simulink model "GUAM"  (R2023b)
settings: Solver=FixedStepAuto  StartTime=0.0  StopTime=SimIn.stopTime  FixedStep=Ts  RelTol=1e-3  AbsTol=1e-4  EnableMultiTasking=on
PostLoadFcn:
  | warning('off','sm:sli:setup:compile:LocalSolverNotSupported')
StartFcn:
  | tic
StopFcn:
  | Elapsed_Sim_Time = toc;
model workspace: external: MATLAB File aileronAssembly_DataFile.m (data not in the file)
values from neighbouring files (symbols this model uses):
  Ts = 0.05    [RUNME.m]
undefined symbols (not defined in the file or in its folder): AAC_Param, ang2Ext_coeff, Ki, Ki_scaling_elec, Kp, Leadscrew, motor_friction, R7_sctrl, sigbuilder_block, SimIn, SimPar, sm_aileron_actuator_lib, smiData, X, Y, Z
libraries: sm_lib x608, fl_lib x378, ee_lib x105, nesl_utility x96, simulink x10, eeGeneralControl x7, sh_lib x7, dspstat3 x6, sdl_lib x3, slpidlib x2, aerolibfltsims x2
(part 2 of 22)

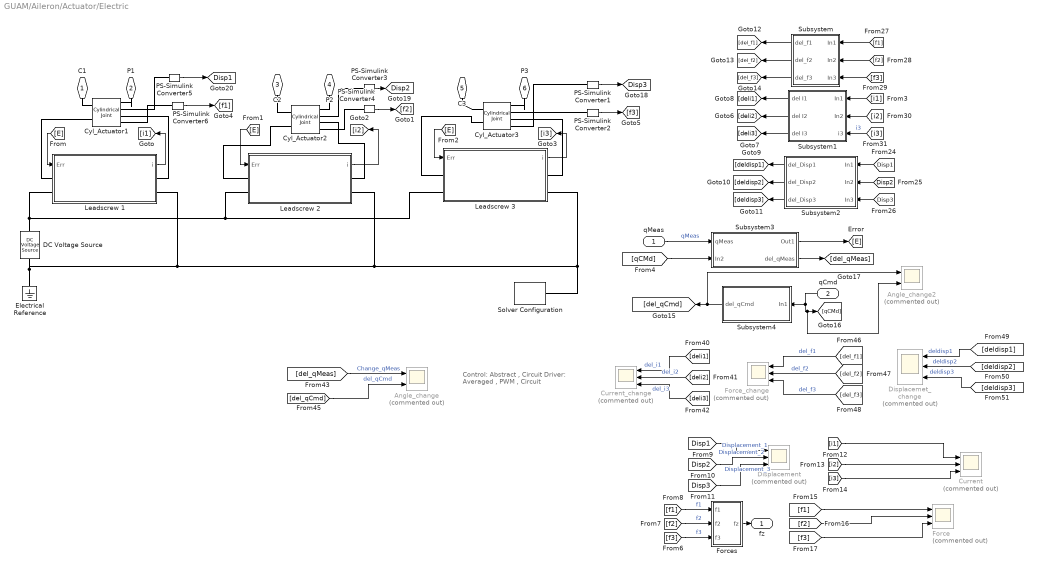
== system GUAM/Aileron/Actuator/Electric ==
  note: Control: Abstract , Circuit
      | Driver: Averaged , PWM , Circuit
  qMeas : Inport
  "qCmd " : Inport  Port=2
  Angle_change : Scope  Commented=on  NumInputPorts=2
  Angle_change2 : Scope  Commented=on  NumInputPorts=2
  Current : Scope  Commented=on  NumInputPorts=3
  Current_change : Scope  Commented=on  NumInputPorts=3
  Cyl_Actuator1 : sm_lib/Joints/Cylindrical Joint  JointMode=Normal  SenseConstraintForce=off  SenseConstraintForceX=off  SenseConstraintForceY=off  SenseConstraintForceZ=off  SenseConstraintTorque=off  SenseConstraintTorqueX=off  SenseConstraintTorqueY=off  SenseConstraintTorqueZ=off  SenseTotalForce=off  SenseTotalForceX=off  SenseTotalForceY=off  SenseTotalForceZ=off  SenseTotalTorque=off  SenseTotalTorqueX=off  SenseTotalTorqueY=off  SenseTotalTorqueZ=off  CompositeWrenchDir=FollowerOnBase  CompositeWrenchFrame=BaseFrame  PzEquilibriumPosition=AAC_Param.Act.El.Spr.l0  PzEquilibriumPositionUnits=m  PzSpringStiffness=AAC_Param.Act.El.Spr.k  PzSpringStiffnessUnits=N/m  PzDampingCoefficient=AAC_Param.Act.El.Spr.b  PzDampingCoefficientUnits=N/(m/s)  PzTorqueActuationMode=InputTorque  PzMotionActuationMode=ComputedMotion  PzSensePosition=on  PzSenseVelocity=on  PzSenseAcceleration=off  PzSenseTorqueForce=on  PzSenseLowerLimitTorqueForce=off  PzSenseUpperLimitTorqueForce=off  PzLowerLimitSpecify=off  PzLowerLimitBound=-1  PzLowerLimitBoundUnits=m  PzLowerLimitStiffness=1e6  PzLowerLimitStiffnessUnits=N/m  PzLowerLimitDamping=1e3  PzLowerLimitDampingUnits=N/(m/s)  PzLowerLimitTransitionRegionWidth=1e-4  PzLowerLimitTransitionRegionWidthUnits=m  PzUpperLimitSpecify=off  PzUpperLimitBound=1  PzUpperLimitBoundUnits=m  PzUpperLimitStiffness=1e6  PzUpperLimitStiffnessUnits=N/m  PzUpperLimitDamping=1e3  PzUpperLimitDampingUnits=N/(m/s)  PzUpperLimitTransitionRegionWidth=1e-4  PzUpperLimitTransitionRegionWidthUnits=m  PzPositionTargetSpecify=on  PzPositionTargetPriority=Low  PzPositionTargetValue=smiData.CylindricalJoint(3).Pz.Pos  PzPositionTargetValueUnits=m  PzVelocityTargetSpecify=off  PzVelocityTargetPriority=High  PzVelocityTargetValue=0  PzVelocityTargetValueUnits=m/s  RzEquilibriumPosition=0  RzEquilibriumPositionUnits=rad  RzSpringStiffness=0  RzSpringStiffnessUnits=N*m/rad  RzDampingCoefficient=0  RzDampingCoefficientUnits=N*m/(rad/s)  RzTorqueActuationMode=NoTorque  RzMotionActuationMode=ComputedMotion  RzSensePosition=off  RzSenseVelocity=off  RzSenseAcceleration=off  RzSenseTorqueForce=off  RzSenseLowerLimitTorqueForce=off  RzSenseUpperLimitTorqueForce=off  RzLowerLimitSpecify=off  RzLowerLimitBound=-90  RzLowerLimitBoundUnits=deg  RzLowerLimitStiffness=1e4  RzLowerLimitStiffnessUnits=N*m/deg  RzLowerLimitDamping=10  RzLowerLimitDampingUnits=N*m/(deg/s)  RzLowerLimitTransitionRegionWidth=0.1  RzLowerLimitTransitionRegionWidthUnits=deg  RzUpperLimitSpecify=off  RzUpperLimitBound=90  RzUpperLimitBoundUnits=deg  RzUpperLimitStiffness=1e4  RzUpperLimitStiffnessUnits=N*m/deg  RzUpperLimitDamping=10  RzUpperLimitDampingUnits=N*m/(deg/s)  RzUpperLimitTransitionRegionWidth=0.1  RzUpperLimitTransitionRegionWidthUnits=deg  RzPositionTargetSpecify=on  RzPositionTargetPriority=Low  RzPositionTargetValue=smiData.CylindricalJoint(3).Rz.Pos  RzPositionTargetValueUnits=deg  RzVelocityTargetSpecify=off  RzVelocityTargetPriority=High  RzVelocityTargetValue=0  RzVelocityTargetValueUnits=deg/s
  Cyl_Actuator2 : sm_lib/Joints/Cylindrical Joint  JointMode=Normal  SenseConstraintForce=off  SenseConstraintForceX=off  SenseConstraintForceY=off  SenseConstraintForceZ=off  SenseConstraintTorque=off  SenseConstraintTorqueX=off  SenseConstraintTorqueY=off  SenseConstraintTorqueZ=off  SenseTotalForce=off  SenseTotalForceX=off  SenseTotalForceY=off  SenseTotalForceZ=off  SenseTotalTorque=off  SenseTotalTorqueX=off  SenseTotalTorqueY=off  SenseTotalTorqueZ=off  CompositeWrenchDir=FollowerOnBase  CompositeWrenchFrame=BaseFrame  PzEquilibriumPosition=AAC_Param.Act.El.Spr.l0  PzEquilibriumPositionUnits=m  PzSpringStiffness=AAC_Param.Act.El.Spr.k  PzSpringStiffnessUnits=N/m  PzDampingCoefficient=AAC_Param.Act.El.Spr.b  PzDampingCoefficientUnits=N/(m/s)  PzTorqueActuationMode=InputTorque  PzMotionActuationMode=ComputedMotion  PzSensePosition=on  PzSenseVelocity=on  PzSenseAcceleration=off  PzSenseTorqueForce=on  PzSenseLowerLimitTorqueForce=off  PzSenseUpperLimitTorqueForce=off  PzLowerLimitSpecify=off  PzLowerLimitBound=-1  PzLowerLimitBoundUnits=m  PzLowerLimitStiffness=1e6  PzLowerLimitStiffnessUnits=N/m  PzLowerLimitDamping=1e3  PzLowerLimitDampingUnits=N/(m/s)  PzLowerLimitTransitionRegionWidth=1e-4  PzLowerLimitTransitionRegionWidthUnits=m  PzUpperLimitSpecify=on  PzUpperLimitBound=1  PzUpperLimitBoundUnits=m  PzUpperLimitStiffness=1e6  PzUpperLimitStiffnessUnits=N/m  PzUpperLimitDamping=1e3  PzUpperLimitDampingUnits=N/(m/s)  PzUpperLimitTransitionRegionWidth=1e-4  PzUpperLimitTransitionRegionWidthUnits=m  PzPositionTargetSpecify=on  PzPositionTargetPriority=Low  PzPositionTargetValue=smiData.CylindricalJoint(2).Pz.Pos  PzPositionTargetValueUnits=m  PzVelocityTargetSpecify=off  PzVelocityTargetPriority=High  PzVelocityTargetValue=0  PzVelocityTargetValueUnits=m/s  RzEquilibriumPosition=0  RzEquilibriumPositionUnits=rad  RzSpringStiffness=0  RzSpringStiffnessUnits=N*m/rad  RzDampingCoefficient=0  RzDampingCoefficientUnits=N*m/(rad/s)  RzTorqueActuationMode=NoTorque  RzMotionActuationMode=ComputedMotion  RzSensePosition=off  RzSenseVelocity=off  RzSenseAcceleration=off  RzSenseTorqueForce=off  RzSenseLowerLimitTorqueForce=off  RzSenseUpperLimitTorqueForce=off  RzLowerLimitSpecify=off  RzLowerLimitBound=-90  RzLowerLimitBoundUnits=deg  RzLowerLimitStiffness=1e4  RzLowerLimitStiffnessUnits=N*m/deg  RzLowerLimitDamping=10  RzLowerLimitDampingUnits=N*m/(deg/s)  RzLowerLimitTransitionRegionWidth=0.1  RzLowerLimitTransitionRegionWidthUnits=deg  RzUpperLimitSpecify=off  RzUpperLimitBound=90  RzUpperLimitBoundUnits=deg  RzUpperLimitStiffness=1e4  RzUpperLimitStiffnessUnits=N*m/deg  RzUpperLimitDamping=10  RzUpperLimitDampingUnits=N*m/(deg/s)  RzUpperLimitTransitionRegionWidth=0.1  RzUpperLimitTransitionRegionWidthUnits=deg  RzPositionTargetSpecify=on  RzPositionTargetPriority=Low  RzPositionTargetValue=smiData.CylindricalJoint(2).Rz.Pos  RzPositionTargetValueUnits=deg  RzVelocityTargetSpecify=off  RzVelocityTargetPriority=High  RzVelocityTargetValue=0  RzVelocityTargetValueUnits=deg/s
  Cyl_Actuator3 : sm_lib/Joints/Cylindrical Joint  JointMode=Normal  SenseConstraintForce=off  SenseConstraintForceX=off  SenseConstraintForceY=off  SenseConstraintForceZ=off  SenseConstraintTorque=off  SenseConstraintTorqueX=off  SenseConstraintTorqueY=off  SenseConstraintTorqueZ=off  SenseTotalForce=off  SenseTotalForceX=off  SenseTotalForceY=off  SenseTotalForceZ=off  SenseTotalTorque=off  SenseTotalTorqueX=off  SenseTotalTorqueY=off  SenseTotalTorqueZ=off  CompositeWrenchDir=FollowerOnBase  CompositeWrenchFrame=BaseFrame  PzEquilibriumPosition=AAC_Param.Act.El.Spr.l0  PzEquilibriumPositionUnits=m  PzSpringStiffness=AAC_Param.Act.El.Spr.k  PzSpringStiffnessUnits=N/m  PzDampingCoefficient=AAC_Param.Act.El.Spr.b  PzDampingCoefficientUnits=N/(m/s)  PzTorqueActuationMode=InputTorque  PzMotionActuationMode=ComputedMotion  PzSensePosition=on  PzSenseVelocity=on  PzSenseAcceleration=off  PzSenseTorqueForce=on  PzSenseLowerLimitTorqueForce=off  PzSenseUpperLimitTorqueForce=off  PzLowerLimitSpecify=off  PzLowerLimitBound=0  PzLowerLimitBoundUnits=m  PzLowerLimitStiffness=1e6  PzLowerLimitStiffnessUnits=N/m  PzLowerLimitDamping=1e3  PzLowerLimitDampingUnits=N/(m/s)  PzLowerLimitTransitionRegionWidth=0.01  PzLowerLimitTransitionRegionWidthUnits=m  PzUpperLimitSpecify=off  PzUpperLimitBound=0.04  PzUpperLimitBoundUnits=m  PzUpperLimitStiffness=1e6  PzUpperLimitStiffnessUnits=N/m  PzUpperLimitDamping=1e3  PzUpperLimitDampingUnits=N/(m/s)  PzUpperLimitTransitionRegionWidth=1e-4  PzUpperLimitTransitionRegionWidthUnits=m  PzPositionTargetSpecify=on  PzPositionTargetPriority=Low  PzPositionTargetValue=smiData.CylindricalJoint(1).Pz.Pos  PzPositionTargetValueUnits=m  PzVelocityTargetSpecify=off  PzVelocityTargetPriority=High  PzVelocityTargetValue=0  PzVelocityTargetValueUnits=m/s  RzEquilibriumPosition=0  RzEquilibriumPositionUnits=rad  RzSpringStiffness=0  RzSpringStiffnessUnits=N*m/rad  RzDampingCoefficient=0  RzDampingCoefficientUnits=N*m/(rad/s)  RzTorqueActuationMode=NoTorque  RzMotionActuationMode=ComputedMotion  RzSensePosition=off  RzSenseVelocity=off  RzSenseAcceleration=off  RzSenseTorqueForce=off  RzSenseLowerLimitTorqueForce=off  RzSenseUpperLimitTorqueForce=off  RzLowerLimitSpecify=off  RzLowerLimitBound=-90  RzLowerLimitBoundUnits=deg  RzLowerLimitStiffness=1e4  RzLowerLimitStiffnessUnits=N*m/deg  RzLowerLimitDamping=10  RzLowerLimitDampingUnits=N*m/(deg/s)  RzLowerLimitTransitionRegionWidth=0.1  RzLowerLimitTransitionRegionWidthUnits=deg  RzUpperLimitSpecify=off  RzUpperLimitBound=90  RzUpperLimitBoundUnits=deg  RzUpperLimitStiffness=1e4  RzUpperLimitStiffnessUnits=N*m/deg  RzUpperLimitDamping=10  RzUpperLimitDampingUnits=N*m/(deg/s)  RzUpperLimitTransitionRegionWidth=0.1  RzUpperLimitTransitionRegionWidthUnits=deg  RzPositionTargetSpecify=on  RzPositionTargetPriority=Low  RzPositionTargetValue=smiData.CylindricalJoint(1).Rz.Pos  RzPositionTargetValueUnits=deg  RzVelocityTargetSpecify=off  RzVelocityTargetPriority=High  RzVelocityTargetValue=0  RzVelocityTargetValueUnits=deg/s
  DC Voltage Source : fl_lib/Electrical/Electrical Sources/DC Voltage Source  v0=24 V
  Displacement : Scope  Commented=on  NumInputPorts=3
  Displacemet_change : Scope  Commented=on  NumInputPorts=3
  Electrical Reference : fl_lib/Electrical/Electrical Elements/Electrical Reference
  Force : Scope  Commented=on  NumInputPorts=3
  Force_change : Scope  Commented=on  NumInputPorts=3
  Forces : Subsystem
  Leadscrew 1 : Subsystem  AncestorBlock=sm_aileron_actuator_lib/Leadscrew  mask{popup_ctrl=Simulink, popup_driver=Averaged}
      mask prompts: popup_ctrl "Controller"; popup_driver "Driver Circuit"
      mask init:
      | if(popup_ctrl == 1)
      |     set_param([gcb '/Control'],'OverrideUsingVariant','Simulink')
      | else
      |     set_param([gcb '/Control'],'OverrideUsingVariant','Circuit')
      | end
      | 
      | if(popup_driver == 3)
      |     set_param([gcb '/Motor Driver'],'OverrideUsingVariant','Circuit')
      | else
      |     set_param([gcb '/Motor Driver'],'OverrideUsingVariant','Abstract')
      |     if(popup_driver == 1)
      |         set_param([gcb '/Motor Driver/Abstract/Controlled PWM Voltage'],'pwm_or_av','2');
      |         set_param([gcb '/Motor Driver/Abstract/H-Bridge'],'pwm_or_av','2');
      |     else
      |         set_param([gcb '/Motor Driver/Abstract/Controlled PWM Voltage'],'pwm_or_av','1');
      |         set_param([gcb '/Motor Driver/Abstract/H-Bridge'],'pwm_or_av','1');
      |     end
      | end
      | 
      | set_param([gcb '/Control'],'Name','Control');
      | set_param([gcb '/Motor Driver'],'Name','Motor Driver');
      mask TypeOptions popup_ctrl: Simulink | Circuit
      mask TypeOptions popup_driver: Averaged | PWM | Circuit
      mask Display:
      | SnC_Char = get_param(gcb,'popup_ctrl');
      | PWM_Char = get_param(gcb,'popup_driver');
      | 
      | try
      |     image(['sm_aileron_actuator_msc' upper(SnC_Char(1)) 'pw' PWM_Char(1) '_IMAGE.png']);
      | catch
      | 
      | end
  Leadscrew 2 : Subsystem  AncestorBlock=sm_aileron_actuator_lib/Leadscrew  mask{popup_ctrl=Simulink, popup_driver=Averaged}
      mask prompts: popup_ctrl "Controller"; popup_driver "Driver Circuit"
      mask init: same as GUAM/Aileron/Actuator/Electric/Leadscrew 1
      mask TypeOptions popup_ctrl: Simulink | Circuit
      mask TypeOptions popup_driver: Averaged | PWM | Circuit
      mask Display:
      | SnC_Char = get_param(gcb,'popup_ctrl');
      | PWM_Char = get_param(gcb,'popup_driver');
      | 
      | try
      |     image(['sm_aileron_actuator_msc' upper(SnC_Char(1)) 'pw' PWM_Char(1) '_IMAGE.png']);
      | catch
      | 
      | end
  Leadscrew 3 : Subsystem  AncestorBlock=sm_aileron_actuator_lib/Leadscrew  mask{popup_ctrl=Simulink, popup_driver=Averaged}
      mask prompts: popup_ctrl "Controller"; popup_driver "Driver Circuit"
      mask init: same as GUAM/Aileron/Actuator/Electric/Leadscrew 1
      mask TypeOptions popup_ctrl: Simulink | Circuit
      mask TypeOptions popup_driver: Averaged | PWM | Circuit
      mask Display:
      | SnC_Char = get_param(gcb,'popup_ctrl');
      | PWM_Char = get_param(gcb,'popup_driver');
      | 
      | try
      |     image(['sm_aileron_actuator_msc' upper(SnC_Char(1)) 'pw' PWM_Char(1) '_IMAGE.png']);
      | catch
      | 
      | end
  PS-Simulink Converter1 : nesl_utility/PS-Simulink Converter  PhysicalDomain=network_engine_domain  SubClassName=ps_output  LeftPortType=input  RightPortType=output  PseudoPeriodic=off  Frequencies=[]  VectorFormat=1-D array  Unit=m  AffineConversion=off
  PS-Simulink Converter2 : nesl_utility/PS-Simulink Converter  PhysicalDomain=network_engine_domain  SubClassName=ps_output  LeftPortType=input  RightPortType=output  PseudoPeriodic=off  Frequencies=[]  VectorFormat=1-D array  Unit=N  AffineConversion=off
  PS-Simulink Converter3 : nesl_utility/PS-Simulink Converter  PhysicalDomain=network_engine_domain  SubClassName=ps_output  LeftPortType=input  RightPortType=output  PseudoPeriodic=off  Frequencies=[]  VectorFormat=1-D array  Unit=m  AffineConversion=off
  PS-Simulink Converter4 : nesl_utility/PS-Simulink Converter  PhysicalDomain=network_engine_domain  SubClassName=ps_output  LeftPortType=input  RightPortType=output  PseudoPeriodic=off  Frequencies=[]  VectorFormat=1-D array  Unit=N  AffineConversion=off
  PS-Simulink Converter5 : nesl_utility/PS-Simulink Converter  PhysicalDomain=network_engine_domain  SubClassName=ps_output  LeftPortType=input  RightPortType=output  PseudoPeriodic=off  Frequencies=[]  VectorFormat=1-D array  Unit=m  AffineConversion=off
  PS-Simulink Converter6 : nesl_utility/PS-Simulink Converter  PhysicalDomain=network_engine_domain  SubClassName=ps_output  LeftPortType=input  RightPortType=output  PseudoPeriodic=off  Frequencies=[]  VectorFormat=1-D array  Unit=N  AffineConversion=off
  Solver Configuration : nesl_utility/Solver Configuration  PhysicalDomain=network_engine_domain  SubClassName=solver  LeftPortType=input  RightPortType=generic  Tones=[]  Harmonics=[]  SimulateNoise=off  Profile=off  UseLocalSampling=off  EnableSwitchedLinearOptims=on  FrequencyDomain=off  UseCCode=off  RelTol=0.001  AbsTol=0.001  MinStep=1e-09  ToWorkspace=off  RevertToSquareIcSolve=off  NumHomotopyIterations=100  PhasorMode=off  PhasorModeNumHarmonics=1  ConsistencySolver=NEWTON_XTOL_AFTER_FTOL  IndexReductionMethod=DerivativeReplacement  DoDC=off  ResidualTolerance=1e-09  ConsistencyTolSource=GLOBAL  ConsistencyAbsTol=0.001  ConsistencyRelTol=0.001  ConsistencyTolFactor=0.0001  UseLocalSolver=off  LocalSolverChoice=NE_BACKWARD_EULER_ADVANCER  ResolveIndetEquations=on  FunctionEvalNumThread=1  LocalSolverSampleTime=0.001  DoFixedCost=off  MaxNonlinIter=3  MaxModeIter=2  ComputeImpulses=off  ImpulseIterations=2  LinearAlgebra=auto  LinearAlgebraNumThread=0  EquationFormulation=NE_TIME_EF  DelaysMemoryBudget=2048  AutomaticFiltering=on  FilteringTimeConstant=0.001  PartitionStorageMethod=AS_NEEDED  PartitionMemoryBudget=1024  PartitionMethod=ROBUST  MultibodyUseLocalSolver=off  MultibodyLocalSolverChoice=ODE1  MultibodyLocalSolverSampleTime=0.001
  Subsystem : Subsystem
  Subsystem1 : Subsystem
  Subsystem2 : Subsystem
  Subsystem3 : Subsystem
  Subsystem4 : Subsystem
  C1 : PMIOPort  Side=Right
  P1 : PMIOPort  Port=2  Side=Right
  C2 : PMIOPort  Port=3  Side=Right
  P2 : PMIOPort  Port=4  Side=Right
  C3 : PMIOPort  Port=5  Side=Right
  P3 : PMIOPort  Port=6  Side=Right
  fz : Outport  VectorParamsAs1DForOutWhenUnconnected=off
  tag scope: Disp1=global, Disp2=global, Disp3=global
  wires:
  [E] -> Leadscrew 1/1(Err)
  [E] -> Leadscrew 2/1(Err)
  [E] -> Leadscrew 3/1(Err)
  Leadscrew 1/1(i) -> [i1]
  Leadscrew 2/1(i) -> [i2]
  Leadscrew 3/1(i) -> [i3]
  [f3] -> Forces/3(f3)  "f3"
  [f2] -> Forces/2(f2)  "f2"
  [f1] -> Forces/1(f1)  "f1"
  Forces/1(fz) -> fz/1
  PS-Simulink Converter4/1 -> [f2]
  PS-Simulink Converter2/1 -> [f3]
  [Disp2] -> Displacement/2  "Displacement_2"
  [Disp1] -> Displacement/1  "Displacement_1"
  [Disp3] -> Displacement/3  "Displacement_3"
  [i2] -> Current/2
  [i3] -> Current/3
  [f2] -> Force/2
  [f3] -> Force/3
  [f1] -> Subsystem/1(In1)
  [f2] -> Subsystem/2(In2)
  [f3] -> Subsystem/3(In3)
  Subsystem/1(del_f1) -> [del_f1]
  Subsystem/2(del_f2) -> [del_f2]
  Subsystem/3(del_f3) -> [del_f3]
  [i1] -> Subsystem1/1(In1)
  [i2] -> Subsystem1/2(In2)
  [i3] -> Subsystem1/3(i3)  "i3"
  Subsystem1/1(del I1) -> [deli1]
  Subsystem1/2(del I2) -> [deli2]
  Subsystem1/3(del I3) -> [deli3]
  [Disp1] -> Subsystem2/1(In1)
  [Disp2] -> Subsystem2/2(In2)
  [Disp3] -> Subsystem2/3(In3)
  Subsystem2/1(del_Disp1) -> [deldisp1]
  Subsystem2/2(del_Disp2) -> [deldisp2]
  Subsystem2/3(del_Disp3) -> [deldisp3]
  PS-Simulink Converter1/1 -> [Disp3]
  PS-Simulink Converter3/1 -> [Disp2]
  PS-Simulink Converter5/1 -> [Disp1]
  [deli1] -> Current_change/1  "del_i1"
  [deli2] -> Current_change/2  "del_i2"
  [deli3] -> Current_change/3  "del_i3"
  qMeas/1 -> Subsystem3/1(qMeas)  "qMeas"
  [qCMd] -> Subsystem3/2(In2)
  Subsystem3/1(Out1) -> [E]
  Subsystem3/2(del_qMeas) -> [del_qMeas]
  "qCmd "/1 -> Angle_change2/2, [qCMd], Subsystem4/1(In1)
  Subsystem4/1(del_qCmd) -> Angle_change2/1, [del_qCmd]
  [del_qMeas] -> Angle_change/1  "Change_qMeas"
  [del_qCmd] -> Angle_change/2  "del_qCmd"
  [del_f1] -> Force_change/1  "del_f1"
  [del_f2] -> Force_change/2  "del_f2"
  [del_f3] -> Force_change/3  "del_f3"
  [deldisp1] -> Displacemet_change/1  "deldisp1"
  [deldisp2] -> Displacemet_change/2  "deldisp2"
  [deldisp3] -> Displacemet_change/3  "deldisp3"
  [f1] -> Force/1
  PS-Simulink Converter6/1 -> [f1]
  [i1] -> Current/1
  connections:
  Leadscrew 3/LConn1 -- Cyl_Actuator3/LConn2
  Cyl_Actuator3/RConn3 -- Leadscrew 3/RConn1
  Leadscrew 2/LConn1 -- Cyl_Actuator2/LConn2
  Leadscrew 1/LConn1 -- Cyl_Actuator1/LConn2
  Leadscrew 1/RConn1 -- Cyl_Actuator1/RConn3
  Cyl_Actuator3/LConn1 -- C3/RConn1
  Cyl_Actuator1/LConn1 -- C1/RConn1
  Cyl_Actuator2/RConn1 -- P2/RConn1
  Cyl_Actuator1/RConn1 -- P1/RConn1
  Cyl_Actuator2/LConn1 -- C2/RConn1
  Electrical Reference/LConn1 -- Solver Configuration/RConn1 -- Leadscrew 3/RConn2 -- Leadscrew 2/RConn2 -- Leadscrew 1/RConn2 -- DC Voltage Source/RConn1
  Leadscrew 2/RConn1 -- Cyl_Actuator2/RConn3
  DC Voltage Source/LConn1 -- Leadscrew 1/LConn2 -- Leadscrew 3/LConn2 -- Leadscrew 2/LConn2
  Cyl_Actuator3/RConn2 -- PS-Simulink Converter1/LConn1
  P3/RConn1 -- Cyl_Actuator3/RConn1
  PS-Simulink Converter2/LConn1 -- Cyl_Actuator3/RConn4
  PS-Simulink Converter4/LConn1 -- Cyl_Actuator2/RConn4
  Cyl_Actuator2/RConn2 -- PS-Simulink Converter3/LConn1
  Cyl_Actuator1/RConn4 -- PS-Simulink Converter6/LConn1
  Cyl_Actuator1/RConn2 -- PS-Simulink Converter5/LConn1
